simulink model "TClabControlDT_R2016a"  (R2016a)
settings: Solver=VariableStepAuto  SolverMode=SingleTasking  StartTime=0.0  StopTime=600  RelTol=1e-3
StartFcn:
  | reset_temp
values from neighbouring files (symbols this model uses):
  Dref = ref-yroom    (= 7)    [setupModelParametersDT.m]    (also in setupModelParametersSat.m = 37)
  ki = 0.1    [setupModelParametersDT.m]    (also in setupModelParametersSat.m)
  kp = 8.75    [setupModelParametersDT.m]    (also in setupModelParametersSat.m)
  P = tf([-tau/2, 1],[tau/2 1])*tf(K,[1 a])    [setupModelParametersDT.m]    (also in setupModelParametersSat.m)
  T = 10    [setupModelParametersDT.m]
undefined symbols (not defined in the file or in its folder): Cd
settings Model: Creator=jamess  LastModifiedBy=jamessaunderson
settings DebuggingCC: SFUnexpectedBacktrackingDiag=error  SFNoUnconditionalDefaultTransitionDiag=error
settings GRTTargetCC: TargetLangStandard=C99 (ISO)
settings ConfigComp: CovMetricSettings=dwe  CovHtmlReporting=off  CovSaveCumulativeToWorkspaceVar=off  CovSaveSingleToWorkspaceVar=off  CovExternalEMLEnable=on

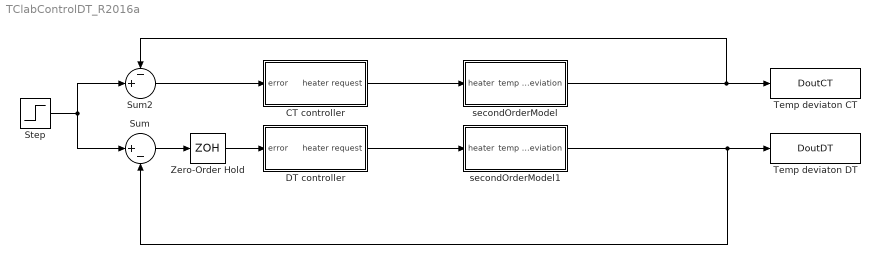
== system TClabControlDT_R2016a ==
  CT controller : Subsystem
  DT controller : Subsystem
  Step : Step  Time=0  After=Dref  SampleTime=0
  Sum : Sum  Inputs=|+-
  Sum2 : Sum  Inputs=-+|
  Temp deviaton CT : ToWorkspace  VariableName=DoutCT  SaveFormat=Timeseries  SampleTime=-1
  Temp deviaton DT : ToWorkspace  VariableName=DoutDT  SaveFormat=Timeseries  SampleTime=-1
  Zero-Order Hold : ZeroOrderHold  SampleTime=T
  secondOrderModel : Subsystem
  secondOrderModel1 : Subsystem
  wires:
  DT controller/1(heater request) -> secondOrderModel1/1(heater)
  Step/1 -> Sum/1, Sum2/2
  secondOrderModel1/1(temp deviation) -> Temp deviaton DT/1, Sum/2
  Sum/1 -> Zero-Order Hold/1
  Sum2/1 -> CT controller/1(error)
  Zero-Order Hold/1 -> DT controller/1(error)
  secondOrderModel/1(temp deviation) -> Temp deviaton CT/1, Sum2/1
  CT controller/1(heater request) -> secondOrderModel/1(heater)

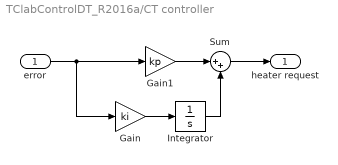
== system TClabControlDT_R2016a/CT controller ==
  error : Inport
  Gain : Gain  Gain=ki
  Gain1 : Gain  Gain=kp
  Integrator : Integrator
  Sum : Sum  Inputs=|++
  heater request : Outport
  wires:
  error/1 -> Gain/1, Gain1/1
  Sum/1 -> heater request/1
  Gain/1 -> Integrator/1
  Gain1/1 -> Sum/1
  Integrator/1 -> Sum/2

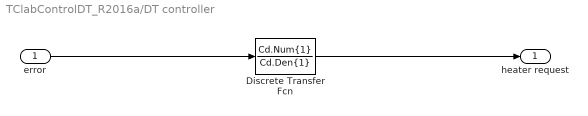
== system TClabControlDT_R2016a/DT controller ==
  error : Inport
  Discrete Transfer Fcn : DiscreteTransferFcn  Numerator=Cd.Num{1}  Denominator=Cd.Den{1}  SampleTime=T
  heater request : Outport
  wires:
  error/1 -> Discrete Transfer Fcn/1
  Discrete Transfer Fcn/1 -> heater request/1

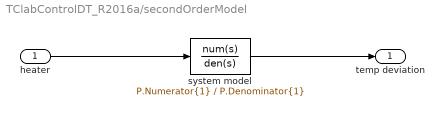
== system TClabControlDT_R2016a/secondOrderModel ==
  heater : Inport
  system model : TransferFcn  Numerator=P.Numerator{1}  Denominator=P.Denominator{1}
  temp deviation : Outport
  wires:
  heater/1 -> system model/1
  system model/1 -> temp deviation/1

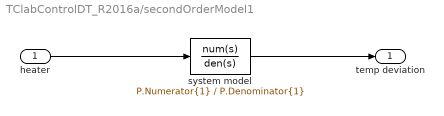
== system TClabControlDT_R2016a/secondOrderModel1 ==
  heater : Inport
  system model : TransferFcn  Numerator=P.Numerator{1}  Denominator=P.Denominator{1}
  temp deviation : Outport
  wires:
  heater/1 -> system model/1
  system model/1 -> temp deviation/1
